simulink model "Multi_Freq_RTC_Etu"  (R2023a)
settings: Solver=ode45  StartTime=0.0  StopTime=10  MaxStep=1e-5  RelTol=1e-3
undefined symbols (not defined in the file or in its folder): XXXX, XXXXX
libraries: dspfdesign x9, simulink_extras x3
settings Model: Creator=p0500439  LastModifiedBy=e2302610
settings SolverCC: AlgebraicLoopSolver=TrustRegion
settings DataIOCC: LimitDataPoints=on  SaveFormat=Array  ReturnWorkspaceOutputs=off
settings OptimizationCC: BlockReduction=off  BooleanDataType=off  LifeSpan=inf
settings DebuggingCC: SaveWithParameterizedLinksMsg=none  UnderspecifiedInitializationDetection=Classic  MergeDetectMultiDrivingBlocksExec=none  SignalResolutionControl=TryResolveAllWithWarning  UnconnectedInputMsg=warning  UnconnectedOutputMsg=warning  UnconnectedLineMsg=warning  SFUnexpectedBacktrackingDiag=warning  SFNoUnconditionalDefaultTransitionDiag=warning  SFExecutionAtInitializationDiag=none  ArithmeticOperatorsInVariantConditions=warning
settings HardwareCC: ProdBitPerPointer=32  ProdBitPerSizeT=32  ProdBitPerPtrDiffT=32  ProdLargestAtomicFloat=None  ProdIntDivRoundTo=Undefined  ProdEndianess=Unspecified  ProdWordSize=32  ProdHWDeviceType=32-bit Generic  TargetUnknown=on
settings ModelReferenceCC: PropagateSignalLabelsOutOfModel=off
settings SFSimCC: SimUseLocalCustomCode=off  CustomCodeUndefinedFunction=UseInterfaceOnly
settings RTWCC: RTWUseLocalCustomCode=off
settings CodeAppCC: StateflowObjectComments=on
settings GRTTargetCC: TargetLangStandard=C89/C90 (ANSI)
settings ConfigComp: CovMetricSettings=dw  CovSaveCumulativeToWorkspaceVar=on  CovSaveSingleToWorkspaceVar=on  CovExternalEMLEnable=off  CovSFcnEnable=off

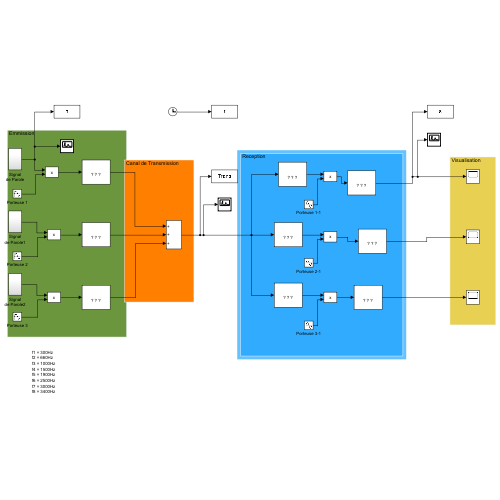
[thumbnail: Simulink's stored preview of the top-level diagram]
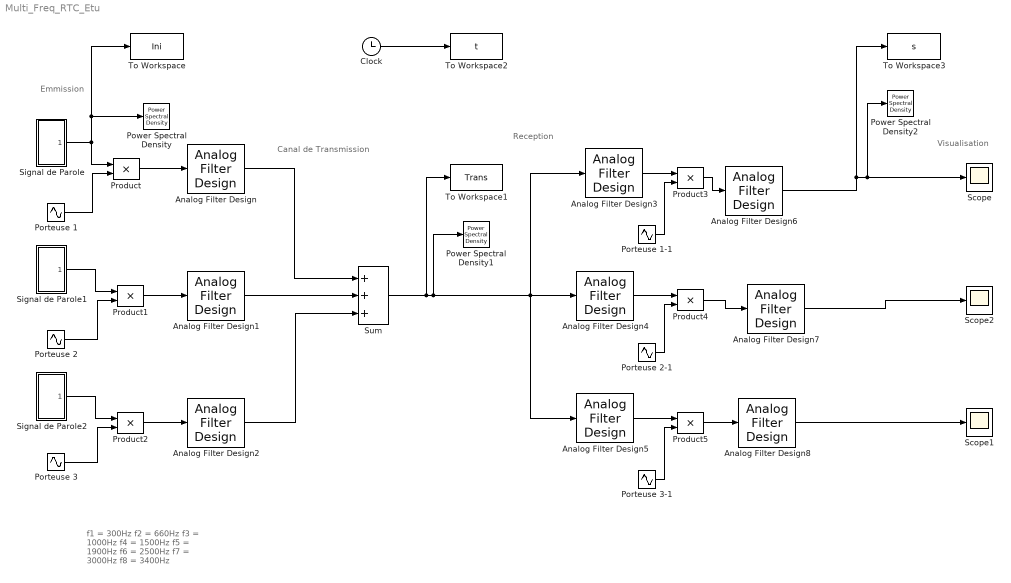
== system Multi_Freq_RTC_Etu ==
  note: Visualisation
  note: Canal de Transmission
  note: Emmission
  note: Reception
  note: f1 = 300Hz
      | f2 = 660Hz
      | f3 = 1000Hz
      | f4 = 1500Hz
      | f5 = 1900Hz
      | f6 = 2500Hz
      | f7 = 3000Hz
      | f8 = 3400Hz
  Analog Filter Design : dspfdesign/Analog Filter Design  method=Chebyshev I  filttype=Lowpass  N=8  Wlo=XXXXXXXXXXXX  Whi=2*pi*8000  Rp=2  Rs=40
  Analog Filter Design1 : dspfdesign/Analog Filter Design  method=Chebyshev I  filttype=Lowpass  N=8  Wlo=XXXXXXXXXXXXX  Whi=2*pi*16000  Rp=2  Rs=40
  Analog Filter Design2 : dspfdesign/Analog Filter Design  method=Chebyshev I  filttype=Lowpass  N=8  Wlo=XXXXXXXXXXXXX  Whi=2*pi*24000  Rp=2  Rs=40
  Analog Filter Design3 : dspfdesign/Analog Filter Design  method=Butterworth  filttype=Lowpass  N=8  Wlo=xXXXXXXXXXXX  Whi=2*pi*8000  Rp=2  Rs=40
  Analog Filter Design4 : dspfdesign/Analog Filter Design  method=Butterworth  filttype=Lowpass  N=8  Wlo=XXXXXXXXXXXX  Whi=2*pi*16000  Rp=2  Rs=40
  Analog Filter Design5 : dspfdesign/Analog Filter Design  method=Butterworth  filttype=Lowpass  N=8  Wlo=XXXXXXXXXXX  Whi=2*pi*24000  Rp=2  Rs=40
  Analog Filter Design6 : dspfdesign/Analog Filter Design  method=Chebyshev I  filttype=Lowpass  N=8  Wlo=XXXXXXXXXXX  Whi=80  Rp=2  Rs=40
  Analog Filter Design7 : dspfdesign/Analog Filter Design  method=Chebyshev I  filttype=Lowpass  N=8  Wlo=XXXXXXXXXXX  Whi=80  Rp=2  Rs=40
  Analog Filter Design8 : dspfdesign/Analog Filter Design  method=Chebyshev I  filttype=Lowpass  N=8  Wlo=XXXXXXXXXXXX  Whi=80  Rp=2  Rs=40
  Clock : Clock
  Porteuse 1 : Sin  Frequency=2*pi*XXXX
  Porteuse 1-1 : Sin  Frequency=2*pi*XXXX
  "Porteuse 2 " : Sin  Frequency=2*pi*XXXX
  Porteuse 2-1 : Sin  Frequency=2*pi*XXXX
  Porteuse 3 : Sin  Frequency=2*pi*XXXX
  Porteuse 3-1 : Sin  Frequency=2*pi*XXXXX
  Power Spectral Density : simulink_extras/Additional Sinks/Power Spectral Density  npts=256  fftpts=1024  HowOften=64  sampleT=1e-4
  Power Spectral Density1 : simulink_extras/Additional Sinks/Power Spectral Density  npts=256  fftpts=1024  HowOften=64  sampleT=1e-5
  Power Spectral Density2 : simulink_extras/Additional Sinks/Power Spectral Density  npts=256  fftpts=1024  HowOften=64  sampleT=1e-4
  Product : Product  InputSameDT=on  RndMeth=Zero  SaturateOnIntegerOverflow=on  SampleTime=1e-6  OutDataTypeStr=Inherit: Same as first input
  Product{1..2,4..5} (4 alike) : Product  InputSameDT=on  RndMeth=Zero  SaturateOnIntegerOverflow=on  OutDataTypeStr=Inherit: Same as first input
  Product3 : Product  InputSameDT=on  RndMeth=Zero  SaturateOnIntegerOverflow=on  SampleTime=1e-6  OutDataTypeStr=Inherit: Same as first input
  Scope : Scope
  Scope1 : Scope
  Scope2 : Scope
  Signal de Parole : Subsystem
  Signal de Parole1 : Subsystem
  Signal de Parole2 : Subsystem
  Sum : Sum  Inputs=+++  InputSameDT=on  SaturateOnIntegerOverflow=on  OutDataTypeStr=Inherit: Same as first input
  To Workspace : ToWorkspace  VariableName=Ini  SampleTime=-1
  To Workspace1 : ToWorkspace  VariableName=Trans  SampleTime=-1
  To Workspace2 : ToWorkspace  VariableName=t  SampleTime=-1
  To Workspace3 : ToWorkspace  VariableName=s  SampleTime=-1
  wires:
  Porteuse 1/1 -> Product/2
  Signal de Parole/1(out_1) -> Product/1, To Workspace/1, Power Spectral Density/1
  "Porteuse 2 "/1 -> Product1/2
  Signal de Parole1/1(out_1) -> Product1/1
  Porteuse 3/1 -> Product2/2
  Signal de Parole2/1(out_1) -> Product2/1
  Sum/1 -> To Workspace1/1, Analog Filter Design5/1, Analog Filter Design4/1, Analog Filter Design3/1, Power Spectral Density1/1
  Product/1 -> Analog Filter Design/1
  Product1/1 -> Analog Filter Design1/1
  Analog Filter Design/1 -> Sum/1
  Analog Filter Design1/1 -> Sum/2
  Product2/1 -> Analog Filter Design2/1
  Analog Filter Design2/1 -> Sum/3
  Product5/1 -> Analog Filter Design8/1
  Product4/1 -> Analog Filter Design7/1
  Product3/1 -> Analog Filter Design6/1
  Analog Filter Design3/1 -> Product3/1
  Porteuse 1-1/1 -> Product3/2
  Analog Filter Design4/1 -> Product4/1
  Porteuse 2-1/1 -> Product4/2
  Analog Filter Design5/1 -> Product5/1
  Porteuse 3-1/1 -> Product5/2
  Analog Filter Design8/1 -> Scope1/1
  Analog Filter Design7/1 -> Scope2/1
  Analog Filter Design6/1 -> To Workspace3/1, Scope/1, Power Spectral Density2/1
  Clock/1 -> To Workspace2/1

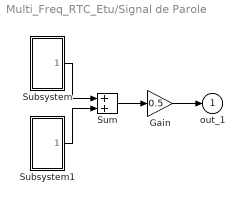
== system Multi_Freq_RTC_Etu/Signal de Parole ==
  Gain : Gain  Gain=0.5  SaturateOnIntegerOverflow=on  OutDataTypeStr=Inherit: Same as input  ParamDataTypeStr=Inherit: Same as input
  Subsystem : Subsystem
  Subsystem1 : Subsystem
  Sum : Sum  InputSameDT=on  SaturateOnIntegerOverflow=on  OutDataTypeStr=Inherit: Same as first input
  out_1 : Outport  VectorParamsAs1DForOutWhenUnconnected=off
  wires:
  Sum/1 -> Gain/1
  Subsystem1/1(out_1) -> Sum/2
  Subsystem/1(out_1) -> Sum/1
  Gain/1 -> out_1/1

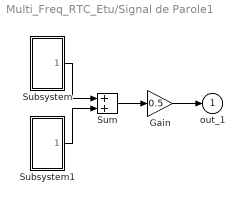
== system Multi_Freq_RTC_Etu/Signal de Parole1 ==
  Gain : Gain  Gain=0.5  SaturateOnIntegerOverflow=on  OutDataTypeStr=Inherit: Same as input  ParamDataTypeStr=Inherit: Same as input
  Subsystem : Subsystem
  Subsystem1 : Subsystem
  Sum : Sum  InputSameDT=on  SaturateOnIntegerOverflow=on  OutDataTypeStr=Inherit: Same as first input
  out_1 : Outport  VectorParamsAs1DForOutWhenUnconnected=off
  wires:
  Sum/1 -> Gain/1
  Subsystem1/1(out_1) -> Sum/2
  Subsystem/1(out_1) -> Sum/1
  Gain/1 -> out_1/1

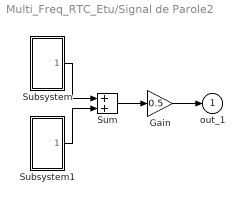
== system Multi_Freq_RTC_Etu/Signal de Parole2 ==
  Gain : Gain  Gain=0.5  SaturateOnIntegerOverflow=on  OutDataTypeStr=Inherit: Same as input  ParamDataTypeStr=Inherit: Same as input
  Subsystem : Subsystem
  Subsystem1 : Subsystem
  Sum : Sum  InputSameDT=on  SaturateOnIntegerOverflow=on  OutDataTypeStr=Inherit: Same as first input
  out_1 : Outport  VectorParamsAs1DForOutWhenUnconnected=off
  wires:
  Sum/1 -> Gain/1
  Subsystem1/1(out_1) -> Sum/2
  Subsystem/1(out_1) -> Sum/1
  Gain/1 -> out_1/1

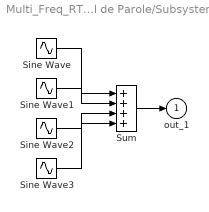
== system Multi_Freq_RTC_Etu/Signal de Parole/Subsystem ==
  Sine Wave : Sin  Amplitude=0.3  Frequency=2*pi*300
  Sine Wave1 : Sin  Amplitude=0.5  Frequency=2*pi*660
  Sine Wave2 : Sin  Amplitude=0.8  Frequency=2*pi*1000
  Sine Wave3 : Sin  Amplitude=0.7  Frequency=2*pi*1500
  Sum : Sum  Inputs=++++  InputSameDT=on  SaturateOnIntegerOverflow=on  OutDataTypeStr=Inherit: Same as first input
  out_1 : Outport  VectorParamsAs1DForOutWhenUnconnected=off
  wires:
  Sine Wave3/1 -> Sum/4
  Sine Wave2/1 -> Sum/3
  Sine Wave1/1 -> Sum/2
  Sine Wave/1 -> Sum/1
  Sum/1 -> out_1/1

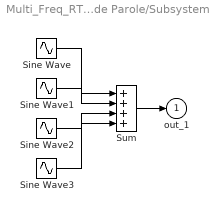
== system Multi_Freq_RTC_Etu/Signal de Parole/Subsystem1 ==
  Sine Wave : Sin  Amplitude=0.3  Frequency=2*pi*1900
  Sine Wave1 : Sin  Amplitude=0.6  Frequency=2*pi*2500
  Sine Wave2 : Sin  Amplitude=0.4  Frequency=2*pi*3000
  Sine Wave3 : Sin  Frequency=2*pi*3400
  Sum : Sum  Inputs=++++  InputSameDT=on  SaturateOnIntegerOverflow=on  OutDataTypeStr=Inherit: Same as first input
  out_1 : Outport  VectorParamsAs1DForOutWhenUnconnected=off
  wires:
  Sum/1 -> out_1/1
  Sine Wave/1 -> Sum/1
  Sine Wave1/1 -> Sum/2
  Sine Wave2/1 -> Sum/3
  Sine Wave3/1 -> Sum/4

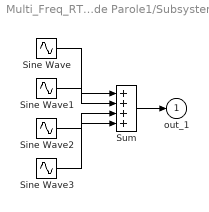
== system Multi_Freq_RTC_Etu/Signal de Parole1/Subsystem ==
  Sine Wave : Sin  Amplitude=0.3  Frequency=2*pi*300
  Sine Wave1 : Sin  Amplitude=0.5  Frequency=2*pi*660
  Sine Wave2 : Sin  Amplitude=0.8  Frequency=2*pi*1000
  Sine Wave3 : Sin  Amplitude=0.7  Frequency=2*pi*1500
  Sum : Sum  Inputs=++++  InputSameDT=on  SaturateOnIntegerOverflow=on  OutDataTypeStr=Inherit: Same as first input
  out_1 : Outport  VectorParamsAs1DForOutWhenUnconnected=off
  wires:
  Sine Wave3/1 -> Sum/4
  Sine Wave2/1 -> Sum/3
  Sine Wave1/1 -> Sum/2
  Sine Wave/1 -> Sum/1
  Sum/1 -> out_1/1

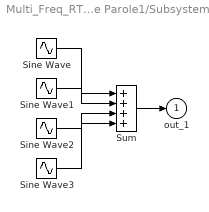
== system Multi_Freq_RTC_Etu/Signal de Parole1/Subsystem1 ==
  Sine Wave : Sin  Amplitude=0.3  Frequency=2*pi*1900
  Sine Wave1 : Sin  Amplitude=0.6  Frequency=2*pi*2500
  Sine Wave2 : Sin  Amplitude=0.4  Frequency=2*pi*3000
  Sine Wave3 : Sin  Frequency=2*pi*3400
  Sum : Sum  Inputs=++++  InputSameDT=on  SaturateOnIntegerOverflow=on  OutDataTypeStr=Inherit: Same as first input
  out_1 : Outport  VectorParamsAs1DForOutWhenUnconnected=off
  wires:
  Sum/1 -> out_1/1
  Sine Wave/1 -> Sum/1
  Sine Wave1/1 -> Sum/2
  Sine Wave2/1 -> Sum/3
  Sine Wave3/1 -> Sum/4

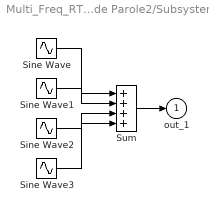
== system Multi_Freq_RTC_Etu/Signal de Parole2/Subsystem ==
  Sine Wave : Sin  Amplitude=0.3  Frequency=2*pi*300
  Sine Wave1 : Sin  Amplitude=0.5  Frequency=2*pi*660
  Sine Wave2 : Sin  Amplitude=0.8  Frequency=2*pi*1000
  Sine Wave3 : Sin  Amplitude=0.7  Frequency=2*pi*1500
  Sum : Sum  Inputs=++++  InputSameDT=on  SaturateOnIntegerOverflow=on  OutDataTypeStr=Inherit: Same as first input
  out_1 : Outport  VectorParamsAs1DForOutWhenUnconnected=off
  wires:
  Sine Wave3/1 -> Sum/4
  Sine Wave2/1 -> Sum/3
  Sine Wave1/1 -> Sum/2
  Sine Wave/1 -> Sum/1
  Sum/1 -> out_1/1

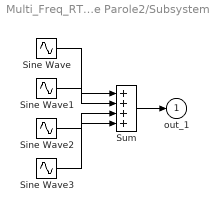
== system Multi_Freq_RTC_Etu/Signal de Parole2/Subsystem1 ==
  Sine Wave : Sin  Amplitude=0.3  Frequency=2*pi*1900
  Sine Wave1 : Sin  Amplitude=0.6  Frequency=2*pi*2500
  Sine Wave2 : Sin  Amplitude=0.4  Frequency=2*pi*3000
  Sine Wave3 : Sin  Frequency=2*pi*3400
  Sum : Sum  Inputs=++++  InputSameDT=on  SaturateOnIntegerOverflow=on  OutDataTypeStr=Inherit: Same as first input
  out_1 : Outport  VectorParamsAs1DForOutWhenUnconnected=off
  wires:
  Sum/1 -> out_1/1
  Sine Wave/1 -> Sum/1
  Sine Wave1/1 -> Sum/2
  Sine Wave2/1 -> Sum/3
  Sine Wave3/1 -> Sum/4
